simulink model "latest_coil"  (R2021b)
settings: Solver=FixedStepAuto  StartTime=-18e-3  StopTime=50e-3  FixedStep=1e-4  RelTol=1e-3
undefined symbols (not defined in the file): X, Y, Z
libraries: sm_lib x28, nesl_utility x9
(part 1 of 5)
settings Model: Creator=teja  LastModifiedBy=teja

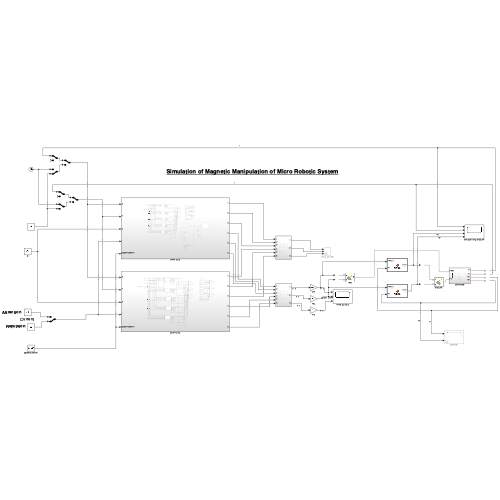
[thumbnail: Simulink's stored preview of the top-level diagram]
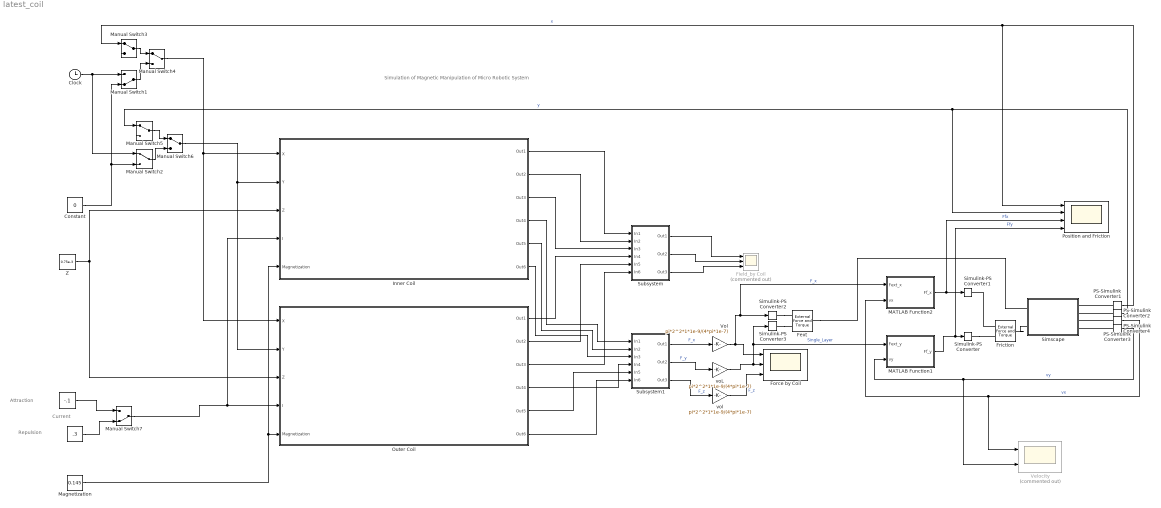
== system latest_coil ==
  note: Current
  note: Attraction
  note: Simulation of Magnetic Manipulation of Micro Robotic System
  note: Repulsion
  " " : Constant  Value=-.1
  "  " : Constant  Value=.3
  Clock : Clock
  Constant : Constant  Value=0
  Fext : sm_lib/Forces and Torques/External Force and Torque  ForceResolutionFrame=World  EnableForceX=on  EnableForceY=on  EnableForceZ=off  EnableForce=off  TorqueResolutionFrame=AttachedFrame  EnableTorqueX=off  EnableTorqueY=off  EnableTorqueZ=off  EnableTorque=off
  Field_by Coil : Scope  Commented=on  NumInputPorts=3
  Force by Coil : Scope  NumInputPorts=3
  Friction : sm_lib/Forces and Torques/External Force and Torque  ForceResolutionFrame=World  EnableForceX=on  EnableForceY=on  EnableForceZ=off  EnableForce=off  TorqueResolutionFrame=AttachedFrame  EnableTorqueX=off  EnableTorqueY=off  EnableTorqueZ=off  EnableTorque=off
  Inner Coil : Subsystem
  MATLAB Function1 : MATLAB Function  TreatAsAtomicUnit=on
  MATLAB Function2 : MATLAB Function  TreatAsAtomicUnit=on
  Magnetization : Constant  Value=0.145
  Manual Switch1 : ManualSwitch  CurrentSetting=0
  Manual Switch{2..6} (5 alike) : ManualSwitch
  Manual Switch7 : ManualSwitch  CurrentSetting=0
  Outer Coil : Subsystem
  PS-Simulink Converter{1..4} (4 alike) : nesl_utility/PS-Simulink Converter  PhysicalDomain=network_engine_domain  SubClassName=ps_output  LeftPortType=input  RightPortType=output  PseudoPeriodic=off  Frequencies=[]  Unit=inherit  AffineConversion=off
      settings: SourceProductBaseCode=PW,SS
  Position and Friction : Scope  NumInputPorts=4
  Simscape : Subsystem
  Simulink-PS Converter{,1..3} (4 alike) : nesl_utility/Simulink-PS Converter  PhysicalDomain=network_engine_domain  SubClassName=ps_input  LeftPortType=input  RightPortType=output  PseudoPeriodic=off  Frequencies=[]  NoiseDistribution=none  NoiseParameters=[]  Unit=1  AffineConversion=off  FilteringAndDerivatives=provide  SimscapeFilterOrder=1  InputFilterTimeConstant=0.001  UdotUserProvided=0
      settings: SourceProductBaseCode=PW,SS
  Subsystem : Subsystem
  Subsystem1 : Subsystem
  Velocity : Scope  Commented=on  NumInputPorts=2
  Vol : Gain  Gain=pi*2^2*1*1e-9/(4*pi*1e-7)
  Z : Constant  Value=0.75e-3
  voL : Gain  Gain=pi*2^2*1*1e-9/(4*pi*1e-7)
  vol : Gain  Gain=pi*2^2*1*1e-9/(4*pi*1e-7)
  wires:
  Constant/1 -> Manual Switch2/2, Manual Switch1/2
  Z/1 -> Outer Coil/3(Z), Inner Coil/3(Z)
  Clock/1 -> Manual Switch2/1, Manual Switch1/1
  Magnetization/1 -> Outer Coil/5(Magnetization), Inner Coil/5(Magnetization)
  Inner Coil/1(Out1) -> Subsystem/1(In1)
  Inner Coil/2(Out2) -> Subsystem/2(In2)
  Inner Coil/3(Out3) -> Subsystem/3(In3)
  Outer Coil/1(Out1) -> Subsystem/4(In4)
  Outer Coil/2(Out2) -> Subsystem/5(In5)
  Outer Coil/3(Out3) -> Subsystem/6(In6)
  Subsystem/1(Out1) -> Field_by Coil/1
  Subsystem/2(Out2) -> Field_by Coil/2
  Subsystem/3(Out3) -> Field_by Coil/3
  Subsystem1/3(Out3) -> vol/1  "F_z"
  Subsystem1/2(Out2) -> voL/1  "F_y"
  Inner Coil/4(Out4) -> Subsystem1/1(In1)
  Inner Coil/5(Out5) -> Subsystem1/2(In2)
  Inner Coil/6(Out6) -> Subsystem1/3(In3)
  Outer Coil/4(Out4) -> Subsystem1/4(In4)
  Outer Coil/5(Out5) -> Subsystem1/5(In5)
  Outer Coil/6(Out6) -> Subsystem1/6(In6)
  Subsystem1/1(Out1) -> Vol/1  "F_x"
  Vol/1 -> MATLAB Function2/1(Fext_x), Simulink-PS Converter2/1, Force by Coil/1  "F_x"
  vol/1 -> Force by Coil/3  "F_z"
  MATLAB Function1/1(Ff_y) -> Position and Friction/4, Simulink-PS Converter/1  "Ffy"
  MATLAB Function2/1(Ff_x) -> Position and Friction/3, Simulink-PS Converter1/1  "Ffx"
  PS-Simulink Converter4/1 -> Velocity/2, MATLAB Function1/2(vy)  "vy"
  PS-Simulink Converter3/1 -> Velocity/1, MATLAB Function2/2(vx)  "vx"
  Manual Switch3/1 -> Manual Switch4/1
  Manual Switch1/1 -> Manual Switch4/2
  Manual Switch4/1 -> Outer Coil/1(X), Inner Coil/1(X)
  PS-Simulink Converter1/1 -> Position and Friction/1, Manual Switch3/1  "x"
  Manual Switch5/1 -> Manual Switch6/1
  Manual Switch2/1 -> Manual Switch6/2
  Manual Switch6/1 -> Outer Coil/2(Y), Inner Coil/2(Y)
  PS-Simulink Converter2/1 -> Position and Friction/2, Manual Switch5/1  "y"
  "  "/1 -> Manual Switch7/2
  " "/1 -> Manual Switch7/1
  Manual Switch7/1 -> Inner Coil/4(I), Outer Coil/4(I)
  voL/1 -> MATLAB Function1/1(Fext_y), Simulink-PS Converter3/1, Force by Coil/2  "Single_Layer"
  connections:
  Fext/RConn1 -- Simscape/LConn1
  Friction/RConn1 -- Simscape/LConn2
  Simulink-PS Converter/RConn1 -- Friction/LConn2
  Friction/LConn1 -- Simulink-PS Converter1/RConn1
  PS-Simulink Converter1/LConn1 -- Simscape/RConn1
  PS-Simulink Converter2/LConn1 -- Simscape/RConn2
  PS-Simulink Converter3/LConn1 -- Simscape/RConn3
  PS-Simulink Converter4/LConn1 -- Simscape/RConn4
  Simulink-PS Converter2/RConn1 -- Fext/LConn1
  Simulink-PS Converter3/RConn1 -- Fext/LConn2

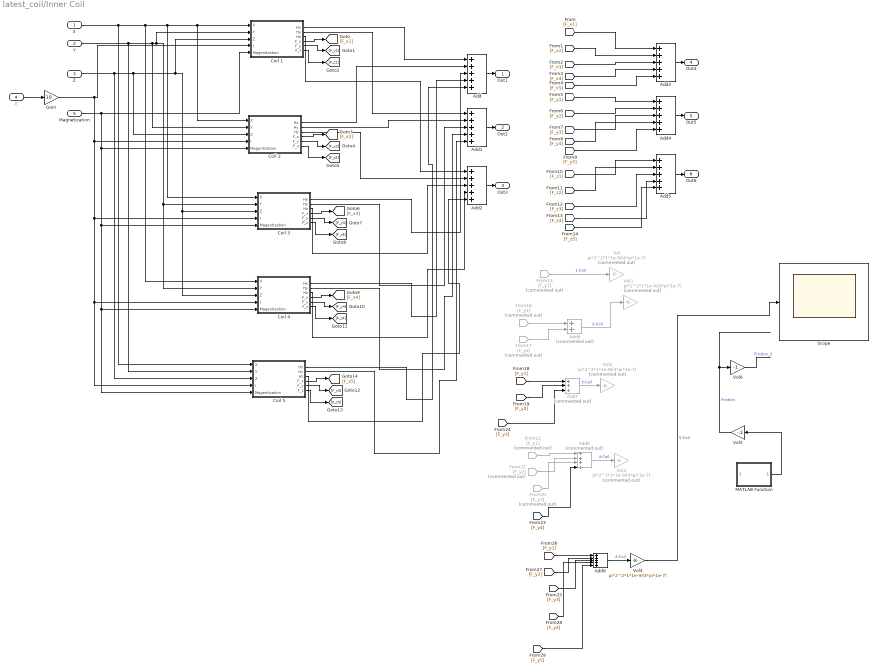
== system latest_coil/Inner Coil ==
  X : Inport
  Y : Inport  Port=2
  Z : Inport  Port=3
  I : Inport  Port=4
  Magnetization : Inport  Port=5
  Add{,1..5,9} (7 alike) : Sum  Inputs=+++++
  Add6 : Sum  Commented=on
  Add7 : Sum  Commented=on  Inputs=+++
  Add8 : Sum  Commented=on  Inputs=++++
  Coil 1 : Subsystem
  Coil 2 : Subsystem
  Coil 3 : Subsystem
  Coil 4 : Subsystem
  Coil 5 : Subsystem
  From15 : From  Commented=on  GotoTag=F_y1
  From16 : From  Commented=on  GotoTag=F_y1
  From17 : From  Commented=on  GotoTag=F_y2
  From20 : From  Commented=on  GotoTag=F_y3
  From21 : From  Commented=on  GotoTag=F_y1
  From22 : From  Commented=on  GotoTag=F_y2
  Gain : Gain  Gain=10
  MATLAB Function : MATLAB Function  TreatAsAtomicUnit=on
  Scope : Scope
  Vol{,1..3} (4 alike) : Gain  Commented=on  Gain=pi*2^2*1*1e-9/(4*pi*1e-7)
  Vol4 : Gain  Gain=pi*2^2*1*1e-9/(4*pi*1e-7)
  Vol5 : Gain  Gain=-.1
  Vol6 : Gain  Gain=-1
  Out1 : Outport
  Out2 : Outport  Port=2
  Out3 : Outport  Port=3
  Out4 : Outport  Port=4
  Out5 : Outport  Port=5
  Out6 : Outport  Port=6
  wires:
  Add2/1 -> Out3/1
  Add1/1 -> Out2/1
  Add/1 -> Out1/1
  Coil 1/1(Hx) -> Add/1
  Coil 1/4(F_x) -> [F_x1]
  Coil 1/5(F_y) -> [F_y1]
  Coil 1/6(F_z) -> [F_z1]
  Coil 1/2(Hy) -> Add1/1
  Coil 1/3(Hz) -> Add2/1
  Coil 2/1(Hx) -> Add/2
  Coil 2/2(Hy) -> Add1/2
  Coil 2/3(Hz) -> Add2/2
  Coil 2/6(F_z) -> [F_z2]
  Coil 2/5(F_y) -> [F_y2]
  Coil 2/4(F_x) -> [F_x2]
  Coil 3/3(Hz) -> Add2/3
  Coil 3/2(Hy) -> Add1/3
  Coil 3/6(F_z) -> [F_z3]
  Coil 3/5(F_y) -> [F_y3]
  Coil 3/4(F_x) -> [F_x3]
  Coil 3/1(Hx) -> Add/3
  Coil 4/1(Hx) -> Add/4
  Coil 4/4(F_x) -> [F_x4]
  Coil 4/5(F_y) -> [F_y4]
  Coil 4/6(F_z) -> [F_z4]
  Coil 4/2(Hy) -> Add1/4
  Coil 4/3(Hz) -> Add2/4
  Coil 5/3(Hz) -> Add2/5
  Coil 5/2(Hy) -> Add1/5
  Coil 5/6(F_z) -> [F_z5]
  Coil 5/5(F_y) -> [F_y5]
  Coil 5/4(F_x) -> [F_x5]
  Magnetization/1 -> Coil 3/5(Magentization), Coil 5/5(Magentization), Coil 4/5(Magentization), Coil 2/5(Magentization), Coil 1/5(Magentization)
  X/1 -> Coil 4/1(X), Coil 3/1(X), Coil 2/1(X), Coil 1/1(X), Coil 5/1(X)
  Coil 5/1(Hx) -> Add/5
  Z/1 -> Coil 5/3(Z), Coil 4/3(Z), Coil 3/3(Z), Coil 1/3(Z), Coil 2/3(Z)
  Y/1 -> Coil 5/2(Y), Coil 4/2(Y), Coil 3/2(Y), Coil 1/2(Y), Coil 2/2(Y)
  Add3/1 -> Out4/1
  Add4/1 -> Out5/1
  Add5/1 -> Out6/1
  [F_x1] -> Add3/1
  [F_y1] -> Add4/1
  [F_x2] -> Add3/2
  [F_x3] -> Add3/3
  [F_x4] -> Add3/4
  [F_x5] -> Add3/5
  [F_y2] -> Add4/2
  [F_y3] -> Add4/3
  [F_y4] -> Add4/4
  [F_y5] -> Add4/5
  [F_z1] -> Add5/1
  [F_z2] -> Add5/2
  [F_z3] -> Add5/3
  [F_z4] -> Add5/4
  [F_z5] -> Add5/5
  From15/1 -> Vol/1  "1-Coil"
  Add6/1 -> Vol1/1  "2-Coil"
  From16/1 -> Add6/1
  From17/1 -> Add6/2
  [F_y2] -> Add7/2
  [F_y1] -> Add7/1
  Add7/1 -> Vol2/1  "3-Coil"
  [F_y4] -> Add8/4
  Add8/1 -> Vol3/1  "4-Coil"
  From21/1 -> Add8/1
  From22/1 -> Add8/2
  [F_y3] -> Add7/3
  From20/1 -> Add8/3
  [F_y3] -> Add9/3
  [F_y2] -> Add9/2
  [F_y1] -> Add9/1
  Add9/1 -> Vol4/1  "4-Coil"
  [F_y4] -> Add9/4
  [F_y5] -> Add9/5
  Vol4/1 -> Scope/1  "5-Coil"
  Vol6/1 -> ?  "Friction_2"
  Vol5/1 -> Vol6/1  "Friction"
  MATLAB Function/1(Force_cy) -> Vol5/1
  I/1 -> Gain/1
  Gain/1 -> Coil 5/4(I), Coil 4/4(I), Coil 3/4(I), Coil 2/4(I), Coil 1/4(I)

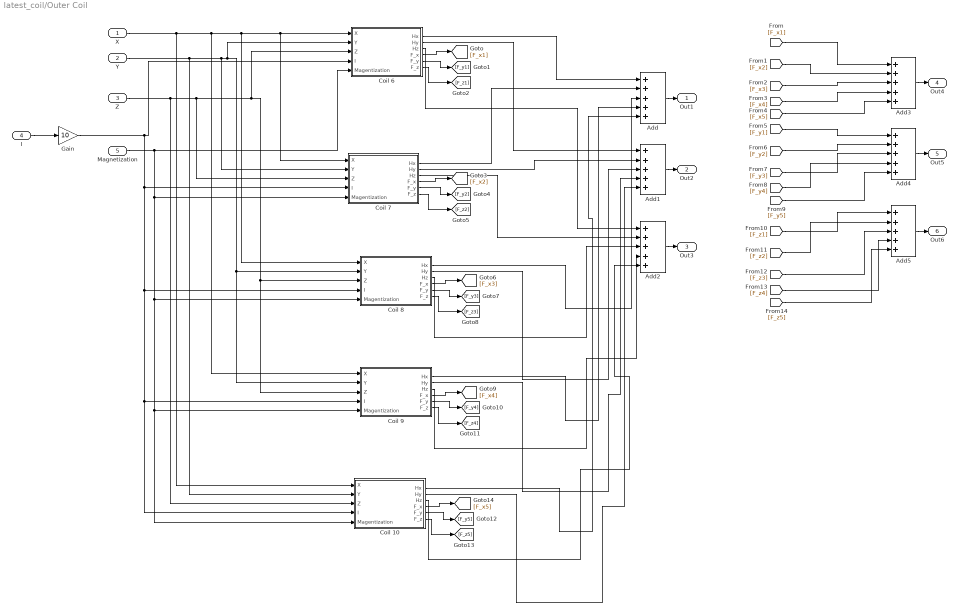
== system latest_coil/Outer Coil ==
  X : Inport
  Y : Inport  Port=2
  Z : Inport  Port=3
  I : Inport  Port=4
  Magnetization : Inport  Port=5
  Add{,1..5} (6 alike) : Sum  Inputs=+++++
  Coil 10 : Subsystem
  Coil 6 : Subsystem
  Coil 7 : Subsystem
  Coil 8 : Subsystem
  Coil 9 : Subsystem
  Gain : Gain  Gain=10
  Out1 : Outport
  Out2 : Outport  Port=2
  Out3 : Outport  Port=3
  Out4 : Outport  Port=4
  Out5 : Outport  Port=5
  Out6 : Outport  Port=6
  wires:
  [F_z5] -> Add5/5
  [F_z4] -> Add5/4
  [F_z3] -> Add5/3
  [F_z2] -> Add5/2
  [F_z1] -> Add5/1
  [F_y5] -> Add4/5
  [F_y4] -> Add4/4
  [F_y3] -> Add4/3
  [F_y2] -> Add4/2
  [F_x5] -> Add3/5
  [F_x4] -> Add3/4
  [F_x3] -> Add3/3
  [F_x2] -> Add3/2
  [F_y1] -> Add4/1
  [F_x1] -> Add3/1
  Add5/1 -> Out6/1
  Add4/1 -> Out5/1
  Add3/1 -> Out4/1
  Y/1 -> Coil 7/2(Y), Coil 6/2(Y), Coil 8/2(Y), Coil 9/2(Y), Coil 10/2(Y)
  Z/1 -> Coil 7/3(Z), Coil 6/3(Z), Coil 8/3(Z), Coil 9/3(Z), Coil 10/3(Z)
  Coil 10/1(Hx) -> Add/5
  X/1 -> Coil 10/1(X), Coil 6/1(X), Coil 7/1(X), Coil 8/1(X), Coil 9/1(X)
  Magnetization/1 -> Coil 6/5(Magentization), Coil 7/5(Magentization), Coil 9/5(Magentization), Coil 10/5(Magentization), Coil 8/5(Magentization)
  Coil 10/4(F_x) -> [F_x5]
  Coil 10/5(F_y) -> [F_y5]
  Coil 10/6(F_z) -> [F_z5]
  Coil 10/2(Hy) -> Add1/5
  Coil 10/3(Hz) -> Add2/5
  Coil 9/3(Hz) -> Add2/4
  Coil 9/2(Hy) -> Add1/4
  Coil 9/6(F_z) -> [F_z4]
  Coil 9/5(F_y) -> [F_y4]
  Coil 9/4(F_x) -> [F_x4]
  Coil 9/1(Hx) -> Add/4
  Coil 8/1(Hx) -> Add/3
  Coil 8/4(F_x) -> [F_x3]
  Coil 8/5(F_y) -> [F_y3]
  Coil 8/6(F_z) -> [F_z3]
  Coil 8/2(Hy) -> Add1/3
  Coil 8/3(Hz) -> Add2/3
  Coil 7/4(F_x) -> [F_x2]
  Coil 7/5(F_y) -> [F_y2]
  Coil 7/6(F_z) -> [F_z2]
  Coil 7/3(Hz) -> Add2/2
  Coil 7/2(Hy) -> Add1/2
  Coil 7/1(Hx) -> Add/2
  Coil 6/3(Hz) -> Add2/1
  Coil 6/2(Hy) -> Add1/1
  Coil 6/6(F_z) -> [F_z1]
  Coil 6/5(F_y) -> [F_y1]
  Coil 6/4(F_x) -> [F_x1]
  Coil 6/1(Hx) -> Add/1
  Add/1 -> Out1/1
  Add1/1 -> Out2/1
  Add2/1 -> Out3/1
  I/1 -> Gain/1
  Gain/1 -> Coil 10/4(I), Coil 9/4(I), Coil 8/4(I), Coil 7/4(I), Coil 6/4(I)

== system latest_coil/Simscape ==
  Base Plate : sm_lib/Body Elements/Brick Solid  GraphicAmbientColor=[0.15 0.15 0.15 1.0]  BasedOnType=Density  BrickDimensions=[100 100 0.15]  BrickDimensionUnits=mm  CenterOfMass=[0 0 0]  CenterOfMassUnits=m  GraphicDiffuseColor=[0.5 0.5 0.5]  Density=1000  DensityUnits=kg/m^3  DoExposeReferenceFrame=off  GraphicEmissiveColor=[0.0 0.0 0.0 1.0]  ExportEntireGeometry=off  SerializedFrames=<Frames><Frame><Id>Frame1</Id><Value><Name>Top</Name><Origin><Source>GeometricFeature</Source><FeatureName>+z surface</FeatureName></Origin><PrimaryAxis><DefinedDirection>+Z</DefinedDirection><Source>ReferenceFrame</Source><SourceDirection>+Z</SourceDirection><FeatureName></FeatureName></PrimaryAxis><SecondaryAxis><DefinedDirection>+X</DefinedDirection><Source>ReferenceFrame</Source><SourceDirection>+X</SourceDirection><FeatureName></FeatureName></SecondaryAxis></Value></Frame></Frames>  MarkerShape=Sphere  MarkerSize=10  GraphicType=FromGeometry  InertiaType=CalculateFromGeometry  Mass=1  MassUnits=kg  MomentsOfInertia=[1 1 1]  MomentsOfInertiaUnits=kg*m^2  GraphicOpacity=1.0  ProductsOfInertia=[0 0 0]  ProductsOfInertiaUnits=kg*m^2  GraphicShininess=75  GraphicSpecularColor=[0.5 0.5 0.5 1.0]  GraphicVisPropType=SimpleVisualProperties
  Bot1 : sm_lib/Body Elements/Cylindrical Solid  GraphicAmbientColor=[0.15 0.15 0.15 1.0]  BasedOnType=Density  CenterOfMass=[0 0 0]  CenterOfMassUnits=m  GraphicDiffuseColor=[0 0 0.5]  CylinderLength=1  CylinderLengthUnits=mm  CylinderRadius=2  CylinderRadiusUnits=mm  Density=7300  DensityUnits=kg/m^3  DoExposeReferenceFrame=on  GraphicEmissiveColor=[0.0 0.0 0.0 1.0]  ExportEntireGeometry=off  SerializedFrames=<Frames><Frame><Id>Frame1</Id><Value><Name>Bottom</Name><Origin><Source>GeometricFeature</Source><FeatureName>bottom surface</FeatureName></Origin><PrimaryAxis><DefinedDirection>+Z</DefinedDirection><Source>ReferenceFrame</Source><SourceDirection>+Z</SourceDirection><FeatureName></FeatureName></PrimaryAxis><SecondaryAxis><DefinedDirection>+X</DefinedDirection><Source>ReferenceFrame</Source><SourceDirection>+X</SourceDirection><FeatureName></FeatureName></SecondaryAxis></Value></Frame></Frames>  MarkerShape=Sphere  MarkerSize=10  GraphicType=FromGeometry  InertiaType=CalculateFromGeometry  Mass=1  MassUnits=kg  MomentsOfInertia=[1 1 1]  MomentsOfInertiaUnits=kg*m^2  GraphicOpacity=1.0  ProductsOfInertia=[0 0 0]  ProductsOfInertiaUnits=kg*m^2  GraphicShininess=75  GraphicSpecularColor=[0.5 0.5 0.5 1.0]  GraphicVisPropType=SimpleVisualProperties
  Brick Solid1 : sm_lib/Body Elements/Brick Solid  GraphicAmbientColor=[0.15 0.15 0.15 1.0]  BasedOnType=Density  BrickDimensions=[8 8 0.5]  BrickDimensionUnits=mm  CenterOfMass=[0 0 0]  CenterOfMassUnits=m  GraphicDiffuseColor=[0 0.5 0]  Density=1000  DensityUnits=kg/m^3  DoExposeReferenceFrame=off  GraphicEmissiveColor=[0.0 0.0 0.0 1.0]  ExportEntireGeometry=off  SerializedFrames=<Frames><Frame><Id>Frame1</Id><Value><Name>base</Name><Origin><Source>GeometricFeature</Source><FeatureName>-z surface</FeatureName></Origin><PrimaryAxis><DefinedDirection>+Z</DefinedDirection><Source>ReferenceFrame</Source><SourceDirection>+Z</SourceDirection><FeatureName></FeatureName></PrimaryAxis><SecondaryAxis><DefinedDirection>+X</DefinedDirection><Source>ReferenceFrame</Source><SourceDirection>+X</SourceDirection><FeatureName></FeatureName></SecondaryAxis></Value></Frame></Frames>  MarkerShape=Sphere  MarkerSize=10  GraphicType=FromGeometry  InertiaType=CalculateFromGeometry  Mass=1  MassUnits=kg  MomentsOfInertia=[1 1 1]  MomentsOfInertiaUnits=kg*m^2  GraphicOpacity=1.0  ProductsOfInertia=[0 0 0]  ProductsOfInertiaUnits=kg*m^2  GraphicShininess=75  GraphicSpecularColor=[0.5 0.5 0.5 1.0]  GraphicVisPropType=SimpleVisualProperties
  Brick Solid{2..9} (8 alike) : sm_lib/Body Elements/Brick Solid  GraphicAmbientColor=[0.15 0.15 0.15 1.0]  BasedOnType=Density  BrickDimensions=[8 8 0.5]  BrickDimensionUnits=mm  CenterOfMass=[0 0 0]  CenterOfMassUnits=m  GraphicDiffuseColor=[0.5 0.5 0]  Density=1000  DensityUnits=kg/m^3  DoExposeReferenceFrame=off  GraphicEmissiveColor=[0.0 0.0 0.0 1.0]  ExportEntireGeometry=off  SerializedFrames=<Frames><Frame><Id>Frame1</Id><Value><Name>base</Name><Origin><Source>GeometricFeature</Source><FeatureName>-z surface</FeatureName></Origin><PrimaryAxis><DefinedDirection>+Z</DefinedDirection><Source>ReferenceFrame</Source><SourceDirection>+Z</SourceDirection><FeatureName></FeatureName></PrimaryAxis><SecondaryAxis><DefinedDirection>+X</DefinedDirection><Source>ReferenceFrame</Source><SourceDirection>+X</SourceDirection><FeatureName></FeatureName></SecondaryAxis></Value></Frame></Frames>  MarkerShape=Sphere  MarkerSize=10  GraphicType=FromGeometry  InertiaType=CalculateFromGeometry  Mass=1  MassUnits=kg  MomentsOfInertia=[1 1 1]  MomentsOfInertiaUnits=kg*m^2  GraphicOpacity=1.0  ProductsOfInertia=[0 0 0]  ProductsOfInertiaUnits=kg*m^2  GraphicShininess=75  GraphicSpecularColor=[0.5 0.5 0.5 1.0]  GraphicVisPropType=SimpleVisualProperties
  Mechanism Configuration : sm_lib/Utilities/Mechanism Configuration  UniformGravity=Constant  GravityVector=[0 0 -9.80665]  GravityUnits=m/s^2  LinearizationDelta=0.001  JointModeTransitionNonlinearIterations=2
  Planar Joint : sm_lib/Joints/Planar Joint  JointMode=Normal  SenseConstraintForce=off  SenseConstraintForceX=off  SenseConstraintForceY=off  SenseConstraintForceZ=off  SenseConstraintTorque=off  SenseConstraintTorqueX=off  SenseConstraintTorqueY=off  SenseConstraintTorqueZ=off  SenseTotalForce=off  SenseTotalForceX=off  SenseTotalForceY=off  SenseTotalForceZ=off  SenseTotalTorque=off  SenseTotalTorqueX=off  SenseTotalTorqueY=off  SenseTotalTorqueZ=off  CompositeWrenchDir=FollowerOnBase  CompositeWrenchFrame=BaseFrame  PxEquilibriumPosition=0  PxEquilibriumPositionUnits=m  PxSpringStiffness=0  PxSpringStiffnessUnits=N/m  PxDampingCoefficient=0  PxDampingCoefficientUnits=N/(m/s)  PxTorqueActuationMode=NoTorque  PxMotionActuationMode=ComputedMotion  PxSensePosition=off  PxSenseVelocity=off  PxSenseAcceleration=off  PxSenseTorqueForce=off  PxSenseLowerLimitTorqueForce=off  PxSenseUpperLimitTorqueForce=off  PxLowerLimitSpecify=off  PxLowerLimitBound=-1  PxLowerLimitBoundUnits=m  PxLowerLimitStiffness=1e6  PxLowerLimitStiffnessUnits=N/m  PxLowerLimitDamping=1e3  PxLowerLimitDampingUnits=N/(m/s)  PxLowerLimitTransitionRegionWidth=1e-4  PxLowerLimitTransitionRegionWidthUnits=m  PxUpperLimitSpecify=off  PxUpperLimitBound=1  PxUpperLimitBoundUnits=m  PxUpperLimitStiffness=1e6  PxUpperLimitStiffnessUnits=N/m  PxUpperLimitDamping=1e3  PxUpperLimitDampingUnits=N/(m/s)  PxUpperLimitTransitionRegionWidth=1e-4  PxUpperLimitTransitionRegionWidthUnits=m  PxPositionTargetSpecify=off  PxPositionTargetPriority=High  PxPositionTargetValue=0  PxPositionTargetValueUnits=m  PxVelocityTargetSpecify=off  PxVelocityTargetPriority=High  PxVelocityTargetValue=0  PxVelocityTargetValueUnits=m/s  PyEquilibriumPosition=0  PyEquilibriumPositionUnits=m  PySpringStiffness=0  PySpringStiffnessUnits=N/m  PyDampingCoefficient=0  PyDampingCoefficientUnits=N/(m/s)  PyTorqueActuationMode=NoTorque  PyMotionActuationMode=ComputedMotion  PySensePosition=off  PySenseVelocity=off  PySenseAcceleration=off  PySenseTorqueForce=off  PySenseLowerLimitTorqueForce=off  PySenseUpperLimitTorqueForce=off  PyLowerLimitSpecify=off  PyLowerLimitBound=-1  PyLowerLimitBoundUnits=m  PyLowerLimitStiffness=1e6  PyLowerLimitStiffnessUnits=N/m  PyLowerLimitDamping=1e3  PyLowerLimitDampingUnits=N/(m/s)  PyLowerLimitTransitionRegionWidth=1e-4  PyLowerLimitTransitionRegionWidthUnits=m  PyUpperLimitSpecify=off  PyUpperLimitBound=1  PyUpperLimitBoundUnits=m  PyUpperLimitStiffness=1e6  PyUpperLimitStiffnessUnits=N/m  PyUpperLimitDamping=1e3  PyUpperLimitDampingUnits=N/(m/s)  PyUpperLimitTransitionRegionWidth=1e-4  PyUpperLimitTransitionRegionWidthUnits=m  PyPositionTargetSpecify=off  PyPositionTargetPriority=High  PyPositionTargetValue=0  PyPositionTargetValueUnits=m  PyVelocityTargetSpecify=off  PyVelocityTargetPriority=High  PyVelocityTargetValue=0  PyVelocityTargetValueUnits=m/s  RzEquilibriumPosition=0  RzEquilibriumPositionUnits=deg  RzSpringStiffness=0  RzSpringStiffnessUnits=N*m/deg  RzDampingCoefficient=0  RzDampingCoefficientUnits=N*m/(deg/s)  RzTorqueActuationMode=NoTorque  RzMotionActuationMode=ComputedMotion  RzSensePosition=off  RzSenseVelocity=off  RzSenseAcceleration=off  RzSenseTorqueForce=off  RzSenseLowerLimitTorqueForce=off  RzSenseUpperLimitTorqueForce=off  RzLowerLimitSpecify=off  RzLowerLimitBound=-90  RzLowerLimitBoundUnits=deg  RzLowerLimitStiffness=1e4  RzLowerLimitStiffnessUnits=N*m/deg  RzLowerLimitDamping=10  RzLowerLimitDampingUnits=N*m/(deg/s)  RzLowerLimitTransitionRegionWidth=0.1  RzLowerLimitTransitionRegionWidthUnits=deg  RzUpperLimitSpecify=off  RzUpperLimitBound=90  RzUpperLimitBoundUnits=deg  RzUpperLimitStiffness=1e4  RzUpperLimitStiffnessUnits=N*m/deg  RzUpperLimitDamping=10  RzUpperLimitDampingUnits=N*m/(deg/s)  RzUpperLimitTransitionRegionWidth=0.1  RzUpperLimitTransitionRegionWidthUnits=deg  RzPositionTargetSpecify=off  RzPositionTargetPriority=High  RzPositionTargetValue=0  RzPositionTargetValueUnits=deg  RzVelocityTargetSpecify=off  RzVelocityTargetPriority=High  RzVelocityTargetValue=0  RzVelocityTargetValueUnits=deg/s
  Rigid Transform1 : sm_lib/Frames and Transforms/Rigid Transform  TranslationMethod=Cartesian  TranslationStandardOffset=0  TranslationLengthUnit=mm  TranslationStandardAxis=+Z  TranslationCartesianOffset=[1 1 0.5]  TranslationROffset=0  TranslationROffsetUnits=m  TranslationZOffset=0  TranslationZOffsetUnits=m  TranslationThetaOffset=0  TranslationThetaOffsetUnits=deg  RotationMethod=AlignedAxes  RotationAngleUnits=deg  RotationStandardAxis=+Z  RotationAngle=0.0  RotationArbitraryAxis=[0 0 1]  FollAlignAxisA=+Y  BaseAlignAxisA=+X  FollAlignAxisB=+Z  BaseAlignAxisB=+Z  RotationSequenceAxes=FollowerAxes  RotationSequence=XYX  RotationSequenceAngles=[0 0 0]  RotationSequenceAnglesUnits=deg  RotationMatrix=[1 0 0; 0 1 0; 0 0 1]
  Rigid Transform10 : sm_lib/Frames and Transforms/Rigid Transform  TranslationMethod=Cartesian  TranslationStandardOffset=0  TranslationLengthUnit=mm  TranslationStandardAxis=+Z  TranslationCartesianOffset=[0 -9 0]  TranslationROffset=0  TranslationROffsetUnits=m  TranslationZOffset=0  TranslationZOffsetUnits=m  TranslationThetaOffset=0  TranslationThetaOffsetUnits=deg  RotationMethod=None  RotationAngleUnits=deg  RotationStandardAxis=+Z  RotationAngle=0.0  RotationArbitraryAxis=[0 0 1]  FollAlignAxisA=+Y  BaseAlignAxisA=+X  FollAlignAxisB=+Z  BaseAlignAxisB=+Z  RotationSequenceAxes=FollowerAxes  RotationSequence=XYX  RotationSequenceAngles=[0 0 0]  RotationSequenceAnglesUnits=deg  RotationMatrix=[1 0 0; 0 1 0; 0 0 1]
  Rigid Transform11 : sm_lib/Frames and Transforms/Rigid Transform  TranslationMethod=Cartesian  TranslationStandardOffset=0  TranslationLengthUnit=mm  TranslationStandardAxis=+Z  TranslationCartesianOffset=[-9 -9 0]  TranslationROffset=0  TranslationROffsetUnits=m  TranslationZOffset=0  TranslationZOffsetUnits=m  TranslationThetaOffset=0  TranslationThetaOffsetUnits=deg  RotationMethod=None  RotationAngleUnits=deg  RotationStandardAxis=+Z  RotationAngle=0.0  RotationArbitraryAxis=[0 0 1]  FollAlignAxisA=+Y  BaseAlignAxisA=+X  FollAlignAxisB=+Z  BaseAlignAxisB=+Z  RotationSequenceAxes=FollowerAxes  RotationSequence=XYX  RotationSequenceAngles=[0 0 0]  RotationSequenceAnglesUnits=deg  RotationMatrix=[1 0 0; 0 1 0; 0 0 1]
  Rigid Transform2 : sm_lib/Frames and Transforms/Rigid Transform  TranslationMethod=None  TranslationStandardOffset=0  TranslationLengthUnit=mm  TranslationStandardAxis=+Z  TranslationCartesianOffset=[0 0 0]  TranslationROffset=0  TranslationROffsetUnits=m  TranslationZOffset=0  TranslationZOffsetUnits=m  TranslationThetaOffset=0  TranslationThetaOffsetUnits=deg  RotationMethod=AlignedAxes  RotationAngleUnits=deg  RotationStandardAxis=+Z  RotationAngle=0.0  RotationArbitraryAxis=[0 0 1]  FollAlignAxisA=+Y  BaseAlignAxisA=+X  FollAlignAxisB=+Z  BaseAlignAxisB=+Z  RotationSequenceAxes=FollowerAxes  RotationSequence=XYX  RotationSequenceAngles=[0 0 0]  RotationSequenceAnglesUnits=deg  RotationMatrix=[1 0 0; 0 1 0; 0 0 1]
  Rigid Transform3 : sm_lib/Frames and Transforms/Rigid Transform  TranslationMethod=Cartesian  TranslationStandardOffset=0  TranslationLengthUnit=mm  TranslationStandardAxis=+Z  TranslationCartesianOffset=[9 0 0]  TranslationROffset=0  TranslationROffsetUnits=m  TranslationZOffset=0  TranslationZOffsetUnits=m  TranslationThetaOffset=0  TranslationThetaOffsetUnits=deg  RotationMethod=None  RotationAngleUnits=deg  RotationStandardAxis=+Z  RotationAngle=0.0  RotationArbitraryAxis=[0 0 1]  FollAlignAxisA=+Y  BaseAlignAxisA=+X  FollAlignAxisB=+Z  BaseAlignAxisB=+Z  RotationSequenceAxes=FollowerAxes  RotationSequence=XYX  RotationSequenceAngles=[0 0 0]  RotationSequenceAnglesUnits=deg  RotationMatrix=[1 0 0; 0 1 0; 0 0 1]
  Rigid Transform4 : sm_lib/Frames and Transforms/Rigid Transform  TranslationMethod=Cartesian  TranslationStandardOffset=0  TranslationLengthUnit=mm  TranslationStandardAxis=+Z  TranslationCartesianOffset=[0 0 0]  TranslationROffset=0  TranslationROffsetUnits=m  TranslationZOffset=0  TranslationZOffsetUnits=m  TranslationThetaOffset=0  TranslationThetaOffsetUnits=deg  RotationMethod=None  RotationAngleUnits=deg  RotationStandardAxis=+Z  RotationAngle=0.0  RotationArbitraryAxis=[0 0 1]  FollAlignAxisA=+Y  BaseAlignAxisA=+X  FollAlignAxisB=+Z  BaseAlignAxisB=+Z  RotationSequenceAxes=FollowerAxes  RotationSequence=XYX  RotationSequenceAngles=[0 0 0]  RotationSequenceAnglesUnits=deg  RotationMatrix=[1 0 0; 0 1 0; 0 0 1]
  Rigid Transform5 : sm_lib/Frames and Transforms/Rigid Transform  TranslationMethod=Cartesian  TranslationStandardOffset=0  TranslationLengthUnit=mm  TranslationStandardAxis=+Z  TranslationCartesianOffset=[-9 0 0]  TranslationROffset=0  TranslationROffsetUnits=m  TranslationZOffset=0  TranslationZOffsetUnits=m  TranslationThetaOffset=0  TranslationThetaOffsetUnits=deg  RotationMethod=None  RotationAngleUnits=deg  RotationStandardAxis=+Z  RotationAngle=0.0  RotationArbitraryAxis=[0 0 1]  FollAlignAxisA=+Y  BaseAlignAxisA=+X  FollAlignAxisB=+Z  BaseAlignAxisB=+Z  RotationSequenceAxes=FollowerAxes  RotationSequence=XYX  RotationSequenceAngles=[0 0 0]  RotationSequenceAnglesUnits=deg  RotationMatrix=[1 0 0; 0 1 0; 0 0 1]
  Rigid Transform6 : sm_lib/Frames and Transforms/Rigid Transform  TranslationMethod=Cartesian  TranslationStandardOffset=0  TranslationLengthUnit=mm  TranslationStandardAxis=+Z  TranslationCartesianOffset=[9 9 0]  TranslationROffset=0  TranslationROffsetUnits=m  TranslationZOffset=0  TranslationZOffsetUnits=m  TranslationThetaOffset=0  TranslationThetaOffsetUnits=deg  RotationMethod=None  RotationAngleUnits=deg  RotationStandardAxis=+Z  RotationAngle=0.0  RotationArbitraryAxis=[0 0 1]  FollAlignAxisA=+Y  BaseAlignAxisA=+X  FollAlignAxisB=+Z  BaseAlignAxisB=+Z  RotationSequenceAxes=FollowerAxes  RotationSequence=XYX  RotationSequenceAngles=[0 0 0]  RotationSequenceAnglesUnits=deg  RotationMatrix=[1 0 0; 0 1 0; 0 0 1]
  Rigid Transform7 : sm_lib/Frames and Transforms/Rigid Transform  TranslationMethod=Cartesian  TranslationStandardOffset=0  TranslationLengthUnit=mm  TranslationStandardAxis=+Z  TranslationCartesianOffset=[0 9 0]  TranslationROffset=0  TranslationROffsetUnits=m  TranslationZOffset=0  TranslationZOffsetUnits=m  TranslationThetaOffset=0  TranslationThetaOffsetUnits=deg  RotationMethod=None  RotationAngleUnits=deg  RotationStandardAxis=+Z  RotationAngle=0.0  RotationArbitraryAxis=[0 0 1]  FollAlignAxisA=+Y  BaseAlignAxisA=+X  FollAlignAxisB=+Z  BaseAlignAxisB=+Z  RotationSequenceAxes=FollowerAxes  RotationSequence=XYX  RotationSequenceAngles=[0 0 0]  RotationSequenceAnglesUnits=deg  RotationMatrix=[1 0 0; 0 1 0; 0 0 1]
  Rigid Transform8 : sm_lib/Frames and Transforms/Rigid Transform  TranslationMethod=Cartesian  TranslationStandardOffset=0  TranslationLengthUnit=mm  TranslationStandardAxis=+Z  TranslationCartesianOffset=[-9 9 0]  TranslationROffset=0  TranslationROffsetUnits=m  TranslationZOffset=0  TranslationZOffsetUnits=m  TranslationThetaOffset=0  TranslationThetaOffsetUnits=deg  RotationMethod=None  RotationAngleUnits=deg  RotationStandardAxis=+Z  RotationAngle=0.0  RotationArbitraryAxis=[0 0 1]  FollAlignAxisA=+Y  BaseAlignAxisA=+X  FollAlignAxisB=+Z  BaseAlignAxisB=+Z  RotationSequenceAxes=FollowerAxes  RotationSequence=XYX  RotationSequenceAngles=[0 0 0]  RotationSequenceAnglesUnits=deg  RotationMatrix=[1 0 0; 0 1 0; 0 0 1]
  Rigid Transform9 : sm_lib/Frames and Transforms/Rigid Transform  TranslationMethod=Cartesian  TranslationStandardOffset=0  TranslationLengthUnit=mm  TranslationStandardAxis=+Z  TranslationCartesianOffset=[9 -9 0]  TranslationROffset=0  TranslationROffsetUnits=m  TranslationZOffset=0  TranslationZOffsetUnits=m  TranslationThetaOffset=0  TranslationThetaOffsetUnits=deg  RotationMethod=None  RotationAngleUnits=deg  RotationStandardAxis=+Z  RotationAngle=0.0  RotationArbitraryAxis=[0 0 1]  FollAlignAxisA=+Y  BaseAlignAxisA=+X  FollAlignAxisB=+Z  BaseAlignAxisB=+Z  RotationSequenceAxes=FollowerAxes  RotationSequence=XYX  RotationSequenceAngles=[0 0 0]  RotationSequenceAnglesUnits=deg  RotationMatrix=[1 0 0; 0 1 0; 0 0 1]
  Solver Configuration : nesl_utility/Solver Configuration  PhysicalDomain=network_engine_domain  SubClassName=solver  LeftPortType=input  RightPortType=generic  Tones=[]  Harmonics=[]  SimulateNoise=off  Profile=off  UseLocalSampling=off  EnableSwitchedLinearOptims=on  FrequencyDomain=off  UseCCode=off  RelTol=0.001  AbsTol=1e-06  MinStep=1e-09  ToWorkspace=off  RevertToSquareIcSolve=off  NumHomotopyIterations=100  PhasorMode=off  PhasorModeNumHarmonics=1  DoDC=off  ResidualTolerance=1e-09  UseLocalSolver=off  LocalSolverChoice=NE_BACKWARD_EULER_ADVANCER  LocalSolverSampleTime=0.001  DoFixedCost=off  MaxNonlinIter=3  MaxModeIter=2  ComputeImpulses=off  ImpulseIterations=2  LinearAlgebra=Sparse  EquationFormulation=NE_TIME_EF  DelaysMemoryBudget=1024  AutomaticFiltering=on  FilteringTimeConstant=0.001  PartitionStorageMethod=AS_NEEDED  PartitionMemoryBudget=1024  PartitionMethod=FAST
      settings: SourceProductBaseCode=PW,SS
  Transform Sensor : sm_lib/Frames and Transforms/Transform Sensor  MeasurementFrame=World  SenseAngle=off  SenseAxis=off  SenseAngle1=off  SenseAngle2=off  SenseAngle3=off  SenseQ=off  SenseR=off  SenseOmegaX=off  SenseOmegaY=off  SenseOmegaZ=off  SenseOmega1=off  SenseOmega2=off  SenseOmega3=off  SenseQDot=off  SenseRDot=off  SenseAlphaX=off  SenseAlphaY=off  SenseAlphaZ=off  SenseAlpha1=off  SenseAlpha2=off  SenseAlpha3=off  SenseQDDot=off  SenseRDDot=off  SenseX=on  SenseY=on  SenseZ=off  SenseRad=off  SenseAzim=off  SenseDist=off  SenseInc=off  SenseXDot=on  SenseYDot=on  SenseZDot=off  SenseRadDot=off  SenseAzimDot=off  SenseDistDot=off  SenseIncDot=off  SenseXDDot=off  SenseYDDot=off  SenseZDDot=off  SenseRadDDot=off  SenseAzimDDot=off  SenseDistDDot=off  SenseIncDDot=off
  World Frame : sm_lib/Frames and Transforms/World Frame
  Fext : PMIOPort  Side=Left
  Ff : PMIOPort  Port=2  Side=Left
  x : PMIOPort  Port=3  Side=Right
  y : PMIOPort  Port=4  Side=Right
  vx : PMIOPort  Port=5  Side=Right
  vy : PMIOPort  Port=6  Side=Right
  connections:
  Rigid Transform1/RConn1 -- Planar Joint/LConn1
  Rigid Transform4/RConn1 -- Brick Solid1/LConn1
  Planar Joint/RConn1 -- Rigid Transform2/LConn1
  Rigid Transform2/RConn1 -- Ff/RConn1 -- Bot1/LConn1
  x/RConn1 -- Transform Sensor/RConn2
  Transform Sensor/RConn3 -- y/RConn1
  vy/RConn1 -- Transform Sensor/RConn5
  vx/RConn1 -- Transform Sensor/RConn4
  Rigid Transform10/LConn1 -- Rigid Transform9/LConn1 -- Rigid Transform11/LConn1 -- Solver Configuration/RConn1 -- Mechanism Configuration/RConn1 -- World Frame/RConn1 -- Rigid Transform1/LConn1 -- Transform Sensor/LConn1 -- Base Plate/LConn1 -- Rigid Transform3/LConn1 -- Rigid Transform4/LConn1 -- Rigid Transform5/LConn1 -- Rigid Transform7/LConn1 -- Rigid Transform8/LConn1 -- Rigid Transform6/LConn1
  Transform Sensor/RConn1 -- Fext/RConn1 -- Bot1/RConn1
  Rigid Transform3/RConn1 -- Brick Solid2/LConn1
  Rigid Transform5/RConn1 -- Brick Solid3/LConn1
  Rigid Transform7/RConn1 -- Brick Solid4/LConn1
  Rigid Transform8/RConn1 -- Brick Solid6/LConn1
  Rigid Transform6/RConn1 -- Brick Solid5/LConn1
  Rigid Transform10/RConn1 -- Brick Solid7/LConn1
  Rigid Transform9/RConn1 -- Brick Solid8/LConn1
  Rigid Transform11/RConn1 -- Brick Solid9/LConn1

== system latest_coil/Subsystem ==
  In1 : Inport
  In2 : Inport  Port=2
  In3 : Inport  Port=3
  In4 : Inport  Port=4
  In5 : Inport  Port=5
  In6 : Inport  Port=6
  Add : Sum
  Add1 : Sum
  Add2 : Sum
  Out1 : Outport
  Out2 : Outport  Port=2
  Out3 : Outport  Port=3
  wires:
  Add2/1 -> Out3/1
  Add/1 -> Out1/1
  Add1/1 -> Out2/1
  In5/1 -> Add1/2
  In4/1 -> Add/2
  In2/1 -> Add1/1
  In6/1 -> Add2/2
  In1/1 -> Add/1
  In3/1 -> Add2/1

== system latest_coil/Subsystem1 ==
  In1 : Inport
  In2 : Inport  Port=2
  In3 : Inport  Port=3
  In4 : Inport  Port=4
  In5 : Inport  Port=5
  In6 : Inport  Port=6
  Add : Sum
  Add1 : Sum
  Add2 : Sum
  Out1 : Outport
  Out2 : Outport  Port=2
  Out3 : Outport  Port=3
  wires:
  In3/1 -> Add2/1
  In1/1 -> Add/1
  In6/1 -> Add2/2
  In2/1 -> Add1/1
  In4/1 -> Add/2
  In5/1 -> Add1/2
  Add1/1 -> Out2/1
  Add/1 -> Out1/1
  Add2/1 -> Out3/1

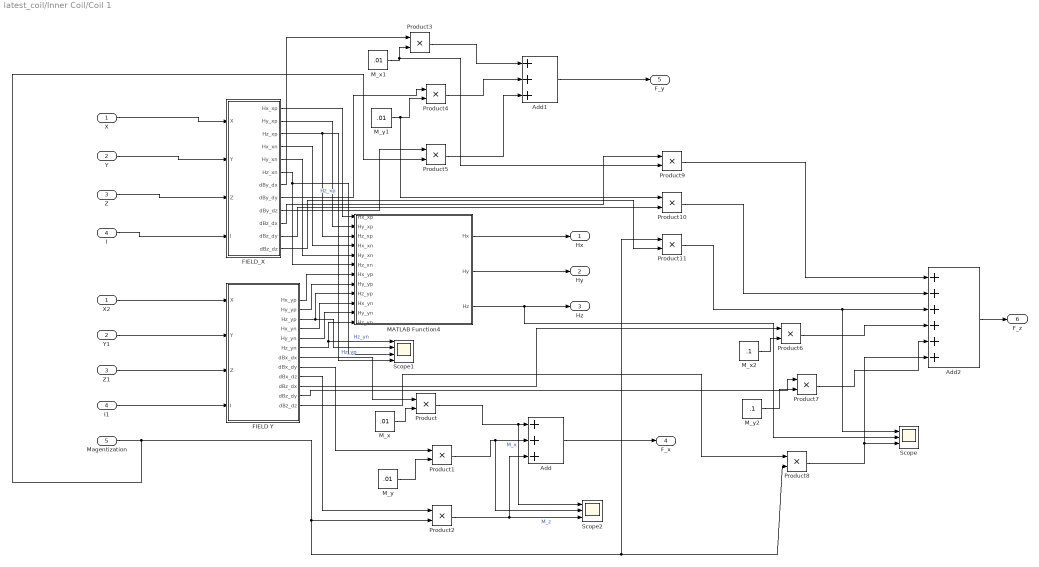
== system latest_coil/Inner Coil/Coil 1 ==
  X : Inport
  Y : Inport  Port=2
  Z : Inport  Port=3
  I : Inport  Port=4
  Magentization : Inport  Port=5
  Add : Sum  Inputs=+++
  Add1 : Sum  Inputs=+++
  Add2 : Sum  Inputs=++++++
  FIELD Y : MATLAB Function  TreatAsAtomicUnit=on
  FIELD_X : MATLAB Function  TreatAsAtomicUnit=on
  I1 : InportShadow  Port=4
  MATLAB Function4 : MATLAB Function  TreatAsAtomicUnit=on
  M_x : Constant  Value=.01
  M_x1 : Constant  Value=.01
  M_x2 : Constant  Value=.1
  M_y : Constant  Value=.01
  M_y1 : Constant  Value=.01
  M_y2 : Constant  Value=.1
  Product{,1..11} (12 alike) : Product
  Scope : Scope  NumInputPorts=3
  Scope1 : Scope  NumInputPorts=4
  Scope2 : Scope  NumInputPorts=3
  X2 : InportShadow
  Y1 : InportShadow  Port=2
  Z1 : InportShadow  Port=3
  Hx : Outport
  Hy : Outport  Port=2
  Hz : Outport  Port=3
  F_x : Outport  Port=4
  F_y : Outport  Port=5
  F_z : Outport  Port=6
  wires:
  MATLAB Function4/3(Hz) -> Scope/2, Hz/1
  X/1 -> FIELD_X/1(X)
  MATLAB Function4/1(Hx) -> Hx/1
  I1/1 -> FIELD Y/4(I)
  FIELD_X/6(Hz_xn) -> Scope1/3, MATLAB Function4/6(Hz_xn)
  Z/1 -> FIELD_X/3(Z)
  FIELD_X/3(Hz_xp) -> Scope1/4, MATLAB Function4/3(Hz_xp)  "Hz_xp"
  MATLAB Function4/2(Hy) -> Hy/1
  FIELD Y/1(Hx_yp) -> MATLAB Function4/7(Hx_yp)
  FIELD Y/4(Hx_yn) -> MATLAB Function4/10(Hx_yn)
  FIELD Y/3(Hz_yp) -> Scope1/2, MATLAB Function4/9(Hz_yp)  "Hz_yp"
  FIELD_X/4(Hx_xn) -> MATLAB Function4/4(Hx_xn)
  FIELD_X/1(Hx_xp) -> MATLAB Function4/1(Hx_xp)
  FIELD Y/2(Hy_yp) -> MATLAB Function4/8(Hy_yp)
  Y/1 -> FIELD_X/2(Y)
  FIELD_X/5(Hy_xn) -> MATLAB Function4/5(Hy_xn)
  FIELD Y/5(Hy_yn) -> MATLAB Function4/11(Hy_yn)
  FIELD Y/6(Hz_yn) -> Scope1/1, MATLAB Function4/12(Hz_yn)  "Hz_yn"
  FIELD_X/2(Hy_xp) -> MATLAB Function4/2(Hy_xp)
  I/1 -> FIELD_X/4(I)
  X2/1 -> FIELD Y/1(X)
  Y1/1 -> FIELD Y/2(Y)
  Z1/1 -> FIELD Y/3(Z)
  M_x/1 -> Product/2
  FIELD Y/7(dBx_dx) -> Product/1
  FIELD Y/8(dBx_dy) -> Product1/1
  M_y/1 -> Product1/2
  FIELD Y/9(dBx_dz) -> Product2/1
  Product/1 -> Scope2/1, Add/1  "M_x"
  Product1/1 -> Scope2/2, Add/2
  Product2/1 -> Scope2/3, Add/3  "M_z"
  Add/1 -> F_x/1
  Add1/1 -> F_y/1
  Product5/1 -> Add1/3
  Product4/1 -> Add1/2
  Product3/1 -> Add1/1
  Magentization/1 -> Product2/2, Product11/1, Product8/2, Product5/2
  FIELD_X/9(dBy_dz) -> Product5/1
  M_y1/1 -> Product10/1, Product4/2
  FIELD_X/7(dBy_dx) -> Product3/1
  Product7/1 -> Add2/5
  Product6/1 -> Add2/4
  M_y2/1 -> Product7/2
  FIELD Y/11(dBz_dy) -> Product7/1
  FIELD Y/10(dBz_dx) -> Product6/1
  M_x2/1 -> Product6/2
  Product8/1 -> Add2/6, Scope/3
  FIELD Y/12(dBz_dz) -> Product8/1
  M_x1/1 -> Product9/2, Product3/2
  FIELD_X/8(dBy_dy) -> Product4/1
  FIELD_X/10(dBz_dx) -> Product9/1
  FIELD_X/11(dBz_dy) -> Product10/2
  FIELD_X/12(dBz_dz) -> Product11/2
  Product9/1 -> Add2/1
  Product10/1 -> Add2/2
  Product11/1 -> Scope/1, Add2/3
  Add2/1 -> F_z/1

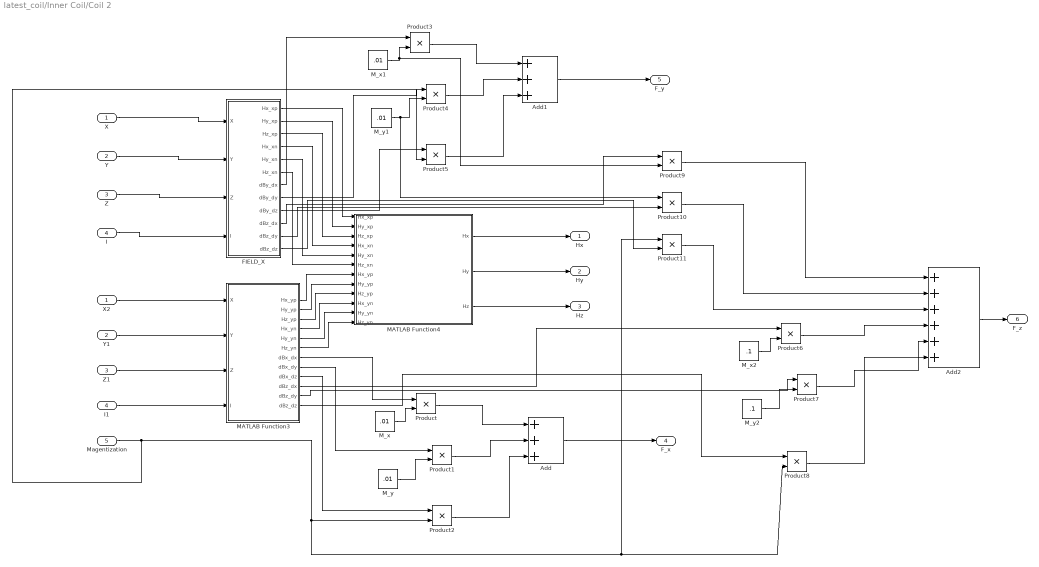
== system latest_coil/Inner Coil/Coil 2 ==
  X : Inport
  Y : Inport  Port=2
  Z : Inport  Port=3
  I : Inport  Port=4
  Magentization : Inport  Port=5
  Add : Sum  Inputs=+++
  Add1 : Sum  Inputs=+++
  Add2 : Sum  Inputs=++++++
  FIELD_X : MATLAB Function  TreatAsAtomicUnit=on
  I1 : InportShadow  Port=4
  MATLAB Function3 : MATLAB Function  TreatAsAtomicUnit=on
  MATLAB Function4 : MATLAB Function  TreatAsAtomicUnit=on
  M_x : Constant  Value=.01
  M_x1 : Constant  Value=.01
  M_x2 : Constant  Value=.1
  M_y : Constant  Value=.01
  M_y1 : Constant  Value=.01
  M_y2 : Constant  Value=.1
  Product{,1..11} (12 alike) : Product
  X2 : InportShadow
  Y1 : InportShadow  Port=2
  Z1 : InportShadow  Port=3
  Hx : Outport
  Hy : Outport  Port=2
  Hz : Outport  Port=3
  F_x : Outport  Port=4
  F_y : Outport  Port=5
  F_z : Outport  Port=6
  wires:
  Add2/1 -> F_z/1
  Product11/1 -> Add2/3
  Product10/1 -> Add2/2
  Product9/1 -> Add2/1
  FIELD_X/12(dBz_dz) -> Product11/2
  FIELD_X/11(dBz_dy) -> Product10/2
  FIELD_X/10(dBz_dx) -> Product9/1
  FIELD_X/8(dBy_dy) -> Product4/1
  M_x1/1 -> Product3/2, Product9/2
  MATLAB Function3/12(dBz_dz) -> Product8/1
  Product8/1 -> Add2/6
  M_x2/1 -> Product6/2
  MATLAB Function3/10(dBz_dx) -> Product6/1
  MATLAB Function3/11(dBz_dy) -> Product7/1
  M_y2/1 -> Product7/2
  Product6/1 -> Add2/4
  Product7/1 -> Add2/5
  FIELD_X/7(dBy_dx) -> Product3/1
  M_y1/1 -> Product4/2, Product10/1
  FIELD_X/9(dBy_dz) -> Product5/1
  Magentization/1 -> Product5/2, Product8/2, Product11/1, Product2/2
  Product3/1 -> Add1/1
  Product4/1 -> Add1/2
  Product5/1 -> Add1/3
  Add1/1 -> F_y/1
  Add/1 -> F_x/1
  Product2/1 -> Add/3
  Product1/1 -> Add/2
  Product/1 -> Add/1
  MATLAB Function3/9(dBx_dz) -> Product2/1
  M_y/1 -> Product1/2
  MATLAB Function3/8(dBx_dy) -> Product1/1
  MATLAB Function3/7(dBx_dx) -> Product/1
  M_x/1 -> Product/2
  Z1/1 -> MATLAB Function3/3(Z)
  Y1/1 -> MATLAB Function3/2(Y)
  X2/1 -> MATLAB Function3/1(X)
  I/1 -> FIELD_X/4(I)
  FIELD_X/2(Hy_xp) -> MATLAB Function4/2(Hy_xp)
  MATLAB Function3/6(Hz_yn) -> MATLAB Function4/12(Hz_yn)
  MATLAB Function3/5(Hy_yn) -> MATLAB Function4/11(Hy_yn)
  FIELD_X/5(Hy_xn) -> MATLAB Function4/5(Hy_xn)
  Y/1 -> FIELD_X/2(Y)
  MATLAB Function3/2(Hy_yp) -> MATLAB Function4/8(Hy_yp)
  FIELD_X/1(Hx_xp) -> MATLAB Function4/1(Hx_xp)
  FIELD_X/4(Hx_xn) -> MATLAB Function4/4(Hx_xn)
  MATLAB Function3/3(Hz_yp) -> MATLAB Function4/9(Hz_yp)
  MATLAB Function3/4(Hx_yn) -> MATLAB Function4/10(Hx_yn)
  MATLAB Function3/1(Hx_yp) -> MATLAB Function4/7(Hx_yp)
  MATLAB Function4/2(Hy) -> Hy/1
  FIELD_X/3(Hz_xp) -> MATLAB Function4/3(Hz_xp)
  Z/1 -> FIELD_X/3(Z)
  FIELD_X/6(Hz_xn) -> MATLAB Function4/6(Hz_xn)
  I1/1 -> MATLAB Function3/4(I)
  MATLAB Function4/1(Hx) -> Hx/1
  X/1 -> FIELD_X/1(X)
  MATLAB Function4/3(Hz) -> Hz/1

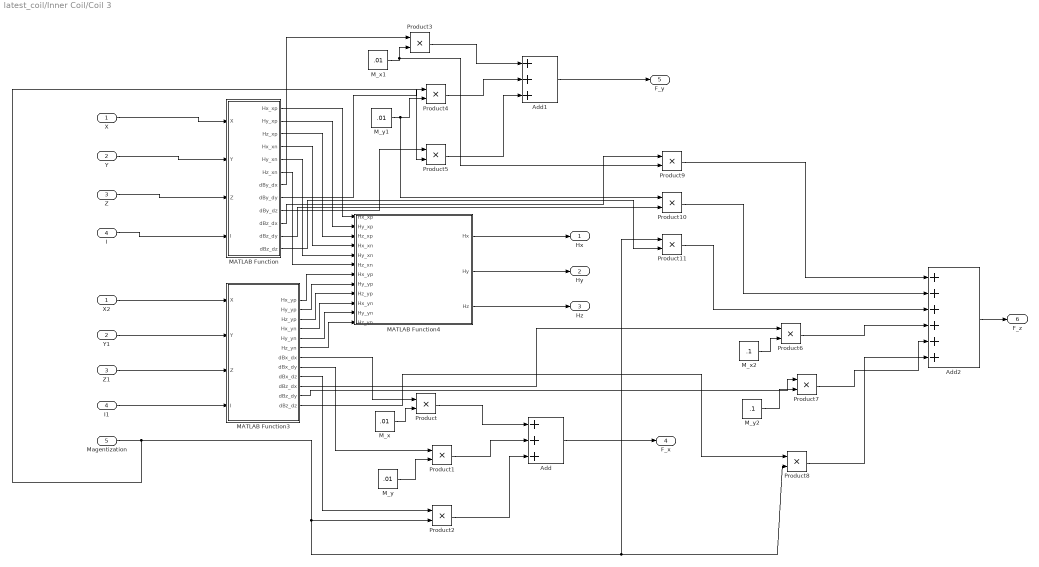
== system latest_coil/Inner Coil/Coil 3 ==
  X : Inport
  Y : Inport  Port=2
  Z : Inport  Port=3
  I : Inport  Port=4
  Magentization : Inport  Port=5
  Add : Sum  Inputs=+++
  Add1 : Sum  Inputs=+++
  Add2 : Sum  Inputs=++++++
  I1 : InportShadow  Port=4
  MATLAB Function : MATLAB Function  TreatAsAtomicUnit=on
  MATLAB Function3 : MATLAB Function  TreatAsAtomicUnit=on
  MATLAB Function4 : MATLAB Function  TreatAsAtomicUnit=on
  M_x : Constant  Value=.01
  M_x1 : Constant  Value=.01
  M_x2 : Constant  Value=.1
  M_y : Constant  Value=.01
  M_y1 : Constant  Value=.01
  M_y2 : Constant  Value=.1
  Product{,1..11} (12 alike) : Product
  X2 : InportShadow
  Y1 : InportShadow  Port=2
  Z1 : InportShadow  Port=3
  Hx : Outport
  Hy : Outport  Port=2
  Hz : Outport  Port=3
  F_x : Outport  Port=4
  F_y : Outport  Port=5
  F_z : Outport  Port=6
  wires:
  Add2/1 -> F_z/1
  Product11/1 -> Add2/3
  Product10/1 -> Add2/2
  Product9/1 -> Add2/1
  MATLAB Function/12(dBz_dz) -> Product11/2
  MATLAB Function/11(dBz_dy) -> Product10/2
  MATLAB Function/10(dBz_dx) -> Product9/1
  MATLAB Function/8(dBy_dy) -> Product4/1
  M_x1/1 -> Product3/2, Product9/2
  MATLAB Function3/12(dBz_dz) -> Product8/1
  Product8/1 -> Add2/6
  M_x2/1 -> Product6/2
  MATLAB Function3/10(dBz_dx) -> Product6/1
  MATLAB Function3/11(dBz_dy) -> Product7/1
  M_y2/1 -> Product7/2
  Product6/1 -> Add2/4
  Product7/1 -> Add2/5
  MATLAB Function/7(dBy_dx) -> Product3/1
  M_y1/1 -> Product4/2, Product10/1
  MATLAB Function/9(dBy_dz) -> Product5/1
  Magentization/1 -> Product5/2, Product8/2, Product11/1, Product2/2
  Product3/1 -> Add1/1
  Product4/1 -> Add1/2
  Product5/1 -> Add1/3
  Add1/1 -> F_y/1
  Add/1 -> F_x/1
  Product2/1 -> Add/3
  Product1/1 -> Add/2
  Product/1 -> Add/1
  MATLAB Function3/9(dBx_dz) -> Product2/1
  M_y/1 -> Product1/2
  MATLAB Function3/8(dBx_dy) -> Product1/1
  MATLAB Function3/7(dBx_dx) -> Product/1
  M_x/1 -> Product/2
  Z1/1 -> MATLAB Function3/3(Z)
  Y1/1 -> MATLAB Function3/2(Y)
  X2/1 -> MATLAB Function3/1(X)
  I/1 -> MATLAB Function/4(I)
  MATLAB Function/2(Hy_xp) -> MATLAB Function4/2(Hy_xp)
  MATLAB Function3/6(Hz_yn) -> MATLAB Function4/12(Hz_yn)
  MATLAB Function3/5(Hy_yn) -> MATLAB Function4/11(Hy_yn)
  MATLAB Function/5(Hy_xn) -> MATLAB Function4/5(Hy_xn)
  Y/1 -> MATLAB Function/2(Y)
  MATLAB Function3/2(Hy_yp) -> MATLAB Function4/8(Hy_yp)
  MATLAB Function/1(Hx_xp) -> MATLAB Function4/1(Hx_xp)
  MATLAB Function/4(Hx_xn) -> MATLAB Function4/4(Hx_xn)
  MATLAB Function3/3(Hz_yp) -> MATLAB Function4/9(Hz_yp)
  MATLAB Function3/4(Hx_yn) -> MATLAB Function4/10(Hx_yn)
  MATLAB Function3/1(Hx_yp) -> MATLAB Function4/7(Hx_yp)
  MATLAB Function4/2(Hy) -> Hy/1
  MATLAB Function/3(Hz_xp) -> MATLAB Function4/3(Hz_xp)
  Z/1 -> MATLAB Function/3(Z)
  MATLAB Function/6(Hz_xn) -> MATLAB Function4/6(Hz_xn)
  I1/1 -> MATLAB Function3/4(I)
  MATLAB Function4/1(Hx) -> Hx/1
  X/1 -> MATLAB Function/1(X)
  MATLAB Function4/3(Hz) -> Hz/1

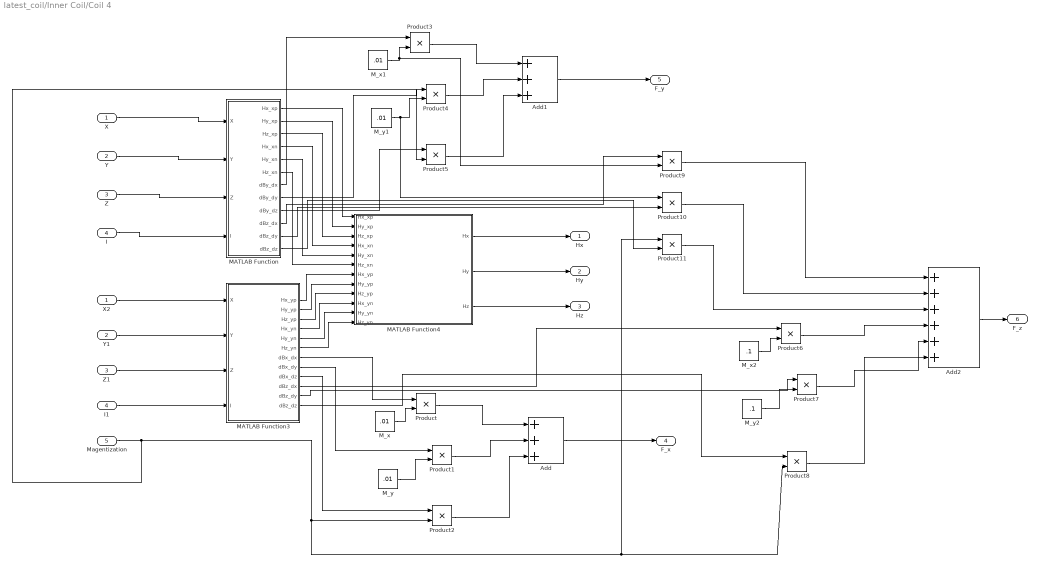
== system latest_coil/Inner Coil/Coil 4 ==
  X : Inport
  Y : Inport  Port=2
  Z : Inport  Port=3
  I : Inport  Port=4
  Magentization : Inport  Port=5
  Add : Sum  Inputs=+++
  Add1 : Sum  Inputs=+++
  Add2 : Sum  Inputs=++++++
  I1 : InportShadow  Port=4
  MATLAB Function : MATLAB Function  TreatAsAtomicUnit=on
  MATLAB Function3 : MATLAB Function  TreatAsAtomicUnit=on
  MATLAB Function4 : MATLAB Function  TreatAsAtomicUnit=on
  M_x : Constant  Value=.01
  M_x1 : Constant  Value=.01
  M_x2 : Constant  Value=.1
  M_y : Constant  Value=.01
  M_y1 : Constant  Value=.01
  M_y2 : Constant  Value=.1
  Product{,1..11} (12 alike) : Product
  X2 : InportShadow
  Y1 : InportShadow  Port=2
  Z1 : InportShadow  Port=3
  Hx : Outport
  Hy : Outport  Port=2
  Hz : Outport  Port=3
  F_x : Outport  Port=4
  F_y : Outport  Port=5
  F_z : Outport  Port=6
  wires:
  MATLAB Function4/3(Hz) -> Hz/1
  X/1 -> MATLAB Function/1(X)
  MATLAB Function4/1(Hx) -> Hx/1
  I1/1 -> MATLAB Function3/4(I)
  MATLAB Function/6(Hz_xn) -> MATLAB Function4/6(Hz_xn)
  Z/1 -> MATLAB Function/3(Z)
  MATLAB Function/3(Hz_xp) -> MATLAB Function4/3(Hz_xp)
  MATLAB Function4/2(Hy) -> Hy/1
  MATLAB Function3/1(Hx_yp) -> MATLAB Function4/7(Hx_yp)
  MATLAB Function3/4(Hx_yn) -> MATLAB Function4/10(Hx_yn)
  MATLAB Function3/3(Hz_yp) -> MATLAB Function4/9(Hz_yp)
  MATLAB Function/4(Hx_xn) -> MATLAB Function4/4(Hx_xn)
  MATLAB Function/1(Hx_xp) -> MATLAB Function4/1(Hx_xp)
  MATLAB Function3/2(Hy_yp) -> MATLAB Function4/8(Hy_yp)
  Y/1 -> MATLAB Function/2(Y)
  MATLAB Function/5(Hy_xn) -> MATLAB Function4/5(Hy_xn)
  MATLAB Function3/5(Hy_yn) -> MATLAB Function4/11(Hy_yn)
  MATLAB Function3/6(Hz_yn) -> MATLAB Function4/12(Hz_yn)
  MATLAB Function/2(Hy_xp) -> MATLAB Function4/2(Hy_xp)
  I/1 -> MATLAB Function/4(I)
  X2/1 -> MATLAB Function3/1(X)
  Y1/1 -> MATLAB Function3/2(Y)
  Z1/1 -> MATLAB Function3/3(Z)
  M_x/1 -> Product/2
  MATLAB Function3/7(dBx_dx) -> Product/1
  MATLAB Function3/8(dBx_dy) -> Product1/1
  M_y/1 -> Product1/2
  MATLAB Function3/9(dBx_dz) -> Product2/1
  Product/1 -> Add/1
  Product1/1 -> Add/2
  Product2/1 -> Add/3
  Add/1 -> F_x/1
  Add1/1 -> F_y/1
  Product5/1 -> Add1/3
  Product4/1 -> Add1/2
  Product3/1 -> Add1/1
  Magentization/1 -> Product2/2, Product11/1, Product8/2, Product5/2
  MATLAB Function/9(dBy_dz) -> Product5/1
  M_y1/1 -> Product10/1, Product4/2
  MATLAB Function/7(dBy_dx) -> Product3/1
  Product7/1 -> Add2/5
  Product6/1 -> Add2/4
  M_y2/1 -> Product7/2
  MATLAB Function3/11(dBz_dy) -> Product7/1
  MATLAB Function3/10(dBz_dx) -> Product6/1
  M_x2/1 -> Product6/2
  Product8/1 -> Add2/6
  MATLAB Function3/12(dBz_dz) -> Product8/1
  M_x1/1 -> Product9/2, Product3/2
  MATLAB Function/8(dBy_dy) -> Product4/1
  MATLAB Function/10(dBz_dx) -> Product9/1
  MATLAB Function/11(dBz_dy) -> Product10/2
  MATLAB Function/12(dBz_dz) -> Product11/2
  Product9/1 -> Add2/1
  Product10/1 -> Add2/2
  Product11/1 -> Add2/3
  Add2/1 -> F_z/1

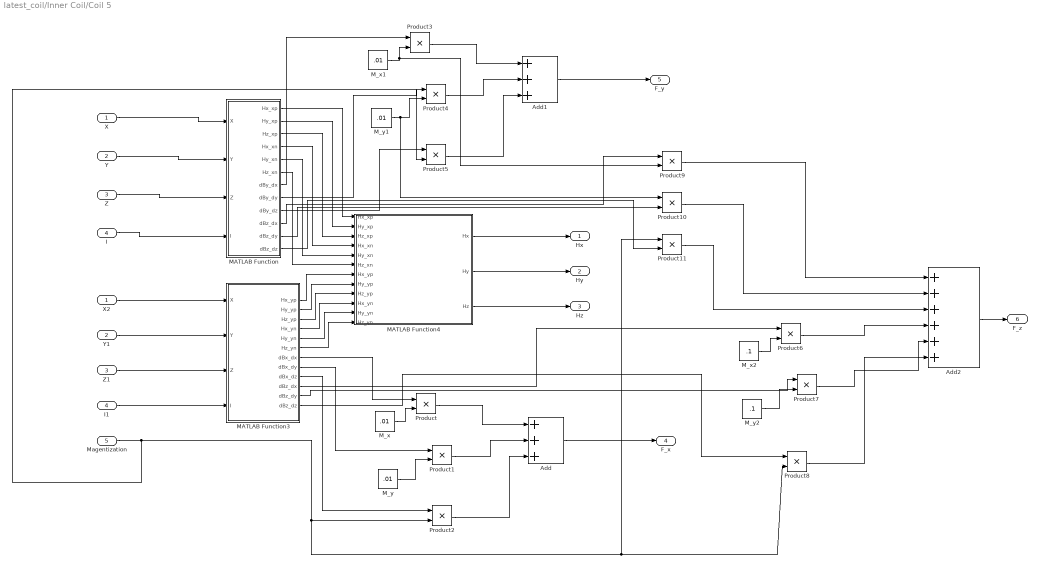
== system latest_coil/Inner Coil/Coil 5 ==
  X : Inport
  Y : Inport  Port=2
  Z : Inport  Port=3
  I : Inport  Port=4
  Magentization : Inport  Port=5
  Add : Sum  Inputs=+++
  Add1 : Sum  Inputs=+++
  Add2 : Sum  Inputs=++++++
  I1 : InportShadow  Port=4
  MATLAB Function : MATLAB Function  TreatAsAtomicUnit=on
  MATLAB Function3 : MATLAB Function  TreatAsAtomicUnit=on
  MATLAB Function4 : MATLAB Function  TreatAsAtomicUnit=on
  M_x : Constant  Value=.01
  M_x1 : Constant  Value=.01
  M_x2 : Constant  Value=.1
  M_y : Constant  Value=.01
  M_y1 : Constant  Value=.01
  M_y2 : Constant  Value=.1
  Product{,1..11} (12 alike) : Product
  X2 : InportShadow
  Y1 : InportShadow  Port=2
  Z1 : InportShadow  Port=3
  Hx : Outport
  Hy : Outport  Port=2
  Hz : Outport  Port=3
  F_x : Outport  Port=4
  F_y : Outport  Port=5
  F_z : Outport  Port=6
  wires:
  Add2/1 -> F_z/1
  Product11/1 -> Add2/3
  Product10/1 -> Add2/2
  Product9/1 -> Add2/1
  MATLAB Function/12(dBz_dz) -> Product11/2
  MATLAB Function/11(dBz_dy) -> Product10/2
  MATLAB Function/10(dBz_dx) -> Product9/1
  MATLAB Function/8(dBy_dy) -> Product4/1
  M_x1/1 -> Product3/2, Product9/2
  MATLAB Function3/12(dBz_dz) -> Product8/1
  Product8/1 -> Add2/6
  M_x2/1 -> Product6/2
  MATLAB Function3/10(dBz_dx) -> Product6/1
  MATLAB Function3/11(dBz_dy) -> Product7/1
  M_y2/1 -> Product7/2
  Product6/1 -> Add2/4
  Product7/1 -> Add2/5
  MATLAB Function/7(dBy_dx) -> Product3/1
  M_y1/1 -> Product4/2, Product10/1
  MATLAB Function/9(dBy_dz) -> Product5/1
  Magentization/1 -> Product5/2, Product8/2, Product11/1, Product2/2
  Product3/1 -> Add1/1
  Product4/1 -> Add1/2
  Product5/1 -> Add1/3
  Add1/1 -> F_y/1
  Add/1 -> F_x/1
  Product2/1 -> Add/3
  Product1/1 -> Add/2
  Product/1 -> Add/1
  MATLAB Function3/9(dBx_dz) -> Product2/1
  M_y/1 -> Product1/2
  MATLAB Function3/8(dBx_dy) -> Product1/1
  MATLAB Function3/7(dBx_dx) -> Product/1
  M_x/1 -> Product/2
  Z1/1 -> MATLAB Function3/3(Z)
  Y1/1 -> MATLAB Function3/2(Y)
  X2/1 -> MATLAB Function3/1(X)
  I/1 -> MATLAB Function/4(I)
  MATLAB Function/2(Hy_xp) -> MATLAB Function4/2(Hy_xp)
  MATLAB Function3/6(Hz_yn) -> MATLAB Function4/12(Hz_yn)
  MATLAB Function3/5(Hy_yn) -> MATLAB Function4/11(Hy_yn)
  MATLAB Function/5(Hy_xn) -> MATLAB Function4/5(Hy_xn)
  Y/1 -> MATLAB Function/2(Y)
  MATLAB Function3/2(Hy_yp) -> MATLAB Function4/8(Hy_yp)
  MATLAB Function/1(Hx_xp) -> MATLAB Function4/1(Hx_xp)
  MATLAB Function/4(Hx_xn) -> MATLAB Function4/4(Hx_xn)
  MATLAB Function3/3(Hz_yp) -> MATLAB Function4/9(Hz_yp)
  MATLAB Function3/4(Hx_yn) -> MATLAB Function4/10(Hx_yn)
  MATLAB Function3/1(Hx_yp) -> MATLAB Function4/7(Hx_yp)
  MATLAB Function4/2(Hy) -> Hy/1
  MATLAB Function/3(Hz_xp) -> MATLAB Function4/3(Hz_xp)
  Z/1 -> MATLAB Function/3(Z)
  MATLAB Function/6(Hz_xn) -> MATLAB Function4/6(Hz_xn)
  I1/1 -> MATLAB Function3/4(I)
  MATLAB Function4/1(Hx) -> Hx/1
  X/1 -> MATLAB Function/1(X)
  MATLAB Function4/3(Hz) -> Hz/1

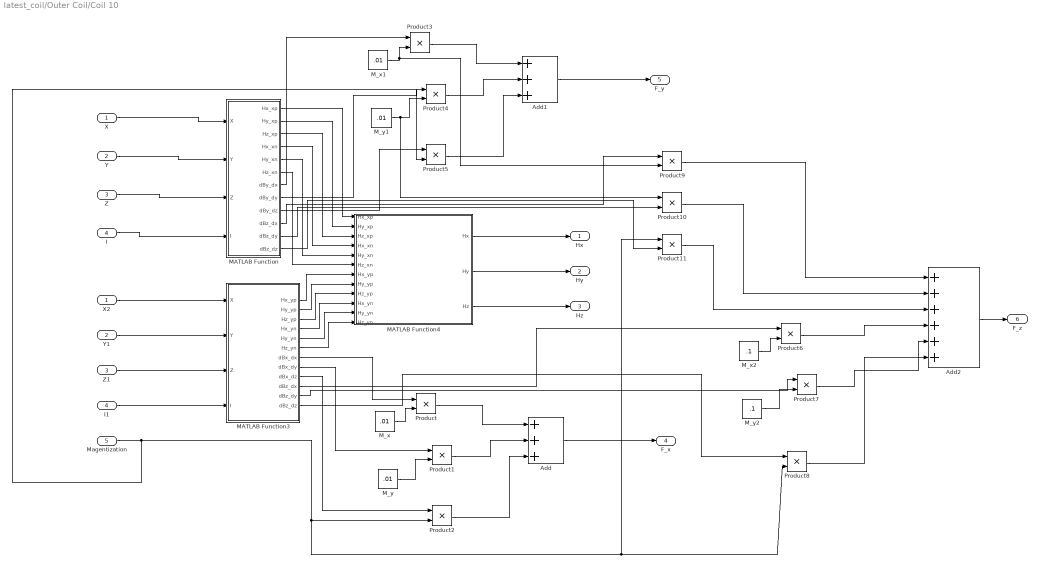
== system latest_coil/Outer Coil/Coil 10 ==
  X : Inport
  Y : Inport  Port=2
  Z : Inport  Port=3
  I : Inport  Port=4
  Magentization : Inport  Port=5
  Add : Sum  Inputs=+++
  Add1 : Sum  Inputs=+++
  Add2 : Sum  Inputs=++++++
  I1 : InportShadow  Port=4
  MATLAB Function : MATLAB Function  TreatAsAtomicUnit=on
  MATLAB Function3 : MATLAB Function  TreatAsAtomicUnit=on
  MATLAB Function4 : MATLAB Function  TreatAsAtomicUnit=on
  M_x : Constant  Value=.01
  M_x1 : Constant  Value=.01
  M_x2 : Constant  Value=.1
  M_y : Constant  Value=.01
  M_y1 : Constant  Value=.01
  M_y2 : Constant  Value=.1
  Product{,1..11} (12 alike) : Product
  X2 : InportShadow
  Y1 : InportShadow  Port=2
  Z1 : InportShadow  Port=3
  Hx : Outport
  Hy : Outport  Port=2
  Hz : Outport  Port=3
  F_x : Outport  Port=4
  F_y : Outport  Port=5
  F_z : Outport  Port=6
  wires:
  MATLAB Function4/3(Hz) -> Hz/1
  X/1 -> MATLAB Function/1(X)
  MATLAB Function4/1(Hx) -> Hx/1
  I1/1 -> MATLAB Function3/4(I)
  MATLAB Function/6(Hz_xn) -> MATLAB Function4/6(Hz_xn)
  Z/1 -> MATLAB Function/3(Z)
  MATLAB Function/3(Hz_xp) -> MATLAB Function4/3(Hz_xp)
  MATLAB Function4/2(Hy) -> Hy/1
  MATLAB Function3/1(Hx_yp) -> MATLAB Function4/7(Hx_yp)
  MATLAB Function3/4(Hx_yn) -> MATLAB Function4/10(Hx_yn)
  MATLAB Function3/3(Hz_yp) -> MATLAB Function4/9(Hz_yp)
  MATLAB Function/4(Hx_xn) -> MATLAB Function4/4(Hx_xn)
  MATLAB Function/1(Hx_xp) -> MATLAB Function4/1(Hx_xp)
  MATLAB Function3/2(Hy_yp) -> MATLAB Function4/8(Hy_yp)
  Y/1 -> MATLAB Function/2(Y)
  MATLAB Function/5(Hy_xn) -> MATLAB Function4/5(Hy_xn)
  MATLAB Function3/5(Hy_yn) -> MATLAB Function4/11(Hy_yn)
  MATLAB Function3/6(Hz_yn) -> MATLAB Function4/12(Hz_yn)
  MATLAB Function/2(Hy_xp) -> MATLAB Function4/2(Hy_xp)
  I/1 -> MATLAB Function/4(I)
  X2/1 -> MATLAB Function3/1(X)
  Y1/1 -> MATLAB Function3/2(Y)
  Z1/1 -> MATLAB Function3/3(Z)
  M_x/1 -> Product/2
  MATLAB Function3/7(dBx_dx) -> Product/1
  MATLAB Function3/8(dBx_dy) -> Product1/1
  M_y/1 -> Product1/2
  MATLAB Function3/9(dBx_dz) -> Product2/1
  Product/1 -> Add/1
  Product1/1 -> Add/2
  Product2/1 -> Add/3
  Add/1 -> F_x/1
  Add1/1 -> F_y/1
  Product5/1 -> Add1/3
  Product4/1 -> Add1/2
  Product3/1 -> Add1/1
  Magentization/1 -> Product2/2, Product11/1, Product8/2, Product5/2
  MATLAB Function/9(dBy_dz) -> Product5/1
  M_y1/1 -> Product10/1, Product4/2
  MATLAB Function/7(dBy_dx) -> Product3/1
  Product7/1 -> Add2/5
  Product6/1 -> Add2/4
  M_y2/1 -> Product7/2
  MATLAB Function3/11(dBz_dy) -> Product7/1
  MATLAB Function3/10(dBz_dx) -> Product6/1
  M_x2/1 -> Product6/2
  Product8/1 -> Add2/6
  MATLAB Function3/12(dBz_dz) -> Product8/1
  M_x1/1 -> Product9/2, Product3/2
  MATLAB Function/8(dBy_dy) -> Product4/1
  MATLAB Function/10(dBz_dx) -> Product9/1
  MATLAB Function/11(dBz_dy) -> Product10/2
  MATLAB Function/12(dBz_dz) -> Product11/2
  Product9/1 -> Add2/1
  Product10/1 -> Add2/2
  Product11/1 -> Add2/3
  Add2/1 -> F_z/1
